simulink model "train_model_nika2"  (R2021b)
settings: Solver=ode4  StartTime=0.0  StopTime=10  FixedStep=0.01  RelTol=1e-3
values from neighbouring files (symbols this model uses):
  g = 9.8    [sis_init.m]
undefined symbols (not defined in the file or in its folder): k, l
libraries: simulink_extras x1
settings Model: Creator=mlx-0  LastModifiedBy=Acer

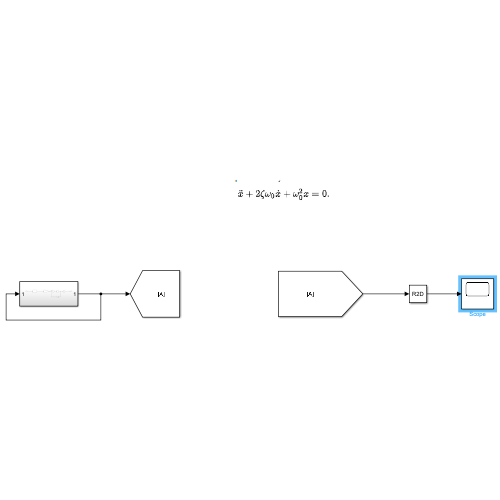
[thumbnail: Simulink's stored preview of the top-level diagram]
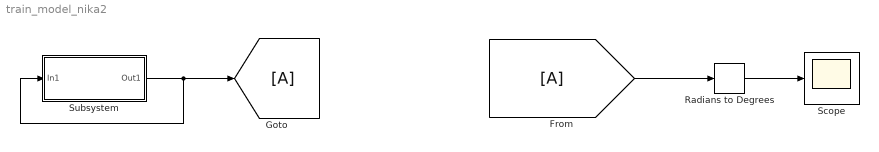
== system train_model_nika2 ==
  Radians to Degrees : simulink_extras/Transformations/Radians to Degrees
  Scope : Scope
  Subsystem : Subsystem
  wires:
  Radians to Degrees/1 -> Scope/1
  Subsystem/1(Out1) -> [A], Subsystem/1(In1)
  [A] -> Radians to Degrees/1

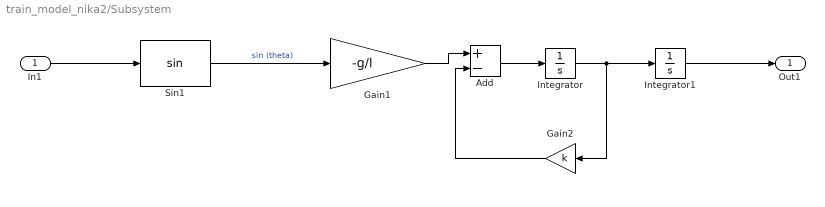
== system train_model_nika2/Subsystem ==
  In1 : Inport  OutDataTypeStr=double
  Add : Sum  Inputs=+-
  Gain1 : Gain  Gain=-g/l
  Gain2 : Gain  Gain=k
  Integrator : Integrator  InitialCondition=0.01
  Integrator1 : Integrator
  Sin1 : Trigonometry
  Out1 : Outport  OutDataTypeStr=double
  wires:
  Gain1/1 -> Add/1
  Gain2/1 -> Add/2
  Integrator/1 -> Gain2/1, Integrator1/1
  Add/1 -> Integrator/1
  Sin1/1 -> Gain1/1  "sin (theta)"
  In1/1 -> Sin1/1
  Integrator1/1 -> Out1/1
